simulink model "Pendulum_LP_linear_w_reg"  (R2024b)
settings: Solver=VariableStepAuto  StartTime=0.0  StopTime=10.0  RelTol=1e-3
values from neighbouring files (symbols this model uses):
  A_upper = [0,  0,                  1,       0 ... (first row only)    [main_LP_w_regulator.m]
  B_upper = [0 ... (first row only)    [main_LP_w_regulator.m]
  K = lqr(A_upper,B_upper,Q,R)    [main_LP_w_regulator.m]
settings Model: Creator=louis  LastModifiedBy=louis

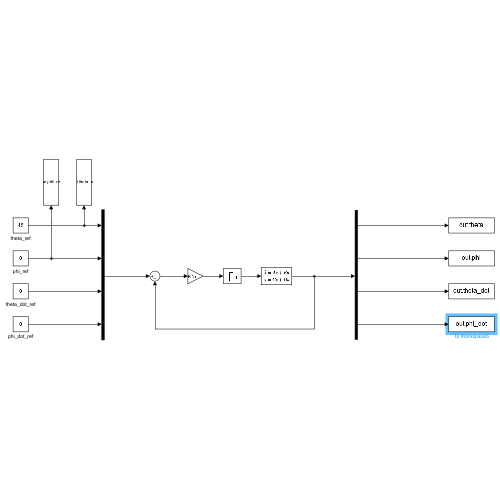
[thumbnail: Simulink's stored preview of the top-level diagram]
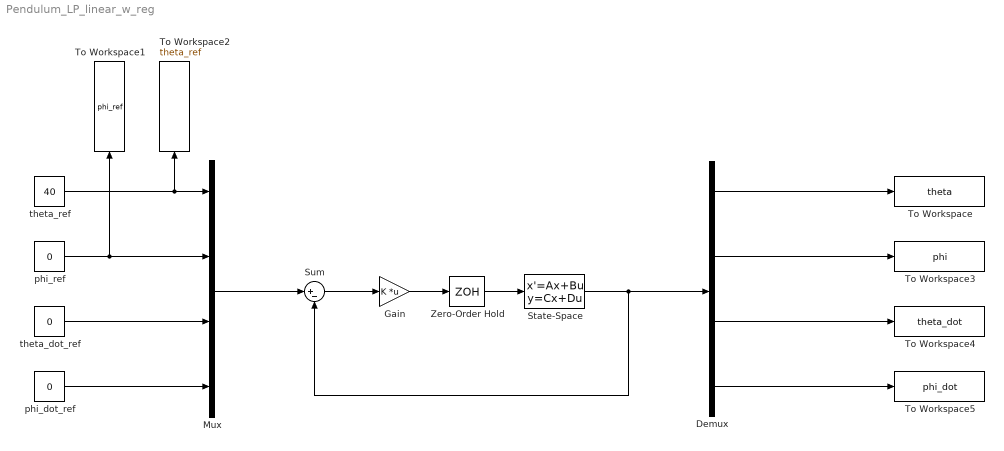
== system Pendulum_LP_linear_w_reg ==
  Demux : Demux
  Gain : Gain  Gain=K  Multiplication=Matrix(K*u)
  Mux : Mux
  State-Space : StateSpace  A=A_upper  B=B_upper  C=eye(4)  D=[0;0;0;0]  InitialCondition=0
  Sum : Sum  Inputs=|+-
  To Workspace : ToWorkspace  VariableName=theta  SaveFormat=Timeseries  SampleTime=-1
  To Workspace1 : ToWorkspace  VariableName=phi_ref  SaveFormat=Timeseries  SampleTime=-1
  To Workspace2 : ToWorkspace  VariableName=theta_ref  SaveFormat=Timeseries  SampleTime=-1
  To Workspace3 : ToWorkspace  VariableName=phi  SaveFormat=Timeseries  SampleTime=-1
  To Workspace4 : ToWorkspace  VariableName=theta_dot  SaveFormat=Timeseries  SampleTime=-1
  To Workspace5 : ToWorkspace  VariableName=phi_dot  SaveFormat=Timeseries  SampleTime=-1
  Zero-Order Hold : ZeroOrderHold  SampleTime=0.01
  phi_dot_ref : Constant  Value=0
  phi_ref : Constant  Value=0
  theta_dot_ref : Constant  Value=0
  theta_ref : Constant  Value=40
  wires:
  theta_dot_ref/1 -> Mux/3
  phi_ref/1 -> To Workspace1/1, Mux/2
  phi_dot_ref/1 -> Mux/4
  theta_ref/1 -> To Workspace2/1, Mux/1
  Gain/1 -> Zero-Order Hold/1
  Zero-Order Hold/1 -> State-Space/1
  Mux/1 -> Sum/1
  State-Space/1 -> Sum/2, Demux/1
  Sum/1 -> Gain/1
  Demux/1 -> To Workspace/1
  Demux/2 -> To Workspace3/1
  Demux/3 -> To Workspace4/1
  Demux/4 -> To Workspace5/1
